simulink model "Michaels_CVModel_fast8"  (R2020a)
settings: Solver=ode23  StartTime=0.0  StopTime=30  RelTol=1e-2  EnableMultiTasking=on
model workspace (MAT data in the model file):
  Eao = 1.88
  Eesla = 0.58
  Eeslvf = 5.2
  Eesra = 0.63
  Eesrvf = 1.75
  Emaxspt = 48.75
  Epa = 0.15
  Epu = 0.04
  Esa = 0.37
  Esv = 0.013
  Evc = 0.03
  GpLV = 0
  GpRR = 11
  GpRV = 0
  GpRsa = 0
  GpV0 = 0
  GsLV = 0.007
  GsRR = 11
  GsRV = 0.022
  GsRsa = -0.05
  GsV0 = 31
  Ka = 4.4
  Lao = 0.0022
  Lav = 0.000354
  Lmt = 7.697e-05
  Lpa = 7.697e-05
  Lpv = 0.0001043
  Ltc = 8.009e-05
  P0la = 0.5
  P0lvf = 0.98
  P0pcd = 0.5
  P0ra = 0.5
  P0rvf = 0.91
  P0spt = 0.46
  PV.AO.p = [0 20 40 60 80 100 120 140 160 180]
  PV.AO.v = [52.2 64.3 81.3 102.1 130 150.7 163.1 173.9 179 183.6]
  PVao = [327.9; 100.9]
  Rao = 0.28
  Rav = 0.02
  Rla2pu = 0.5
  Rmt = 0.01
  Rpa = 0.12
  Rpa_Vals = 0.12
  Rpu = 0.006
  Rpv = 0.02
  Rra = 0.012
  Rsa = 0.74
  Rsv = 0.12
  Rtc = 0.01
  Tc = 1
  Tsys0 = 0.6
  V0la = 30
  V0lvf = 45
  V0pcd = 200
  V0ra = 25
  V0rvf = 50
  V0spt = 10
  Vdla = 15
  Vdlvf = 16
  Vdra = 15
  Vdrvf = 40
  Vdspt = 10
  Vlv0 = 100
  Vperi = 51
  Vrv0 = 105
  Vuao = 260.8
  Vupa = 91
  Vupu = 132
  Vusa = 287.4
  Vusv = 1976.1
  Vuvc = 136.17
  amin = -2
  artBrLVcontConti = []
  artBrLVcontDigi = [0 0 0 0 0 0 0 0 0 0 0 0 ... (240 elements, 1x240)]
  artBrRRConti = []
  artBrRRDigi = [0 0 0 0 0 0 0 0 0 0 1.57142857143 3.14285714286 ... (240 elements, 1x240)]
  artBrRVcontConti = []
  artBrRVcontDigi = [0 0 0 0 0 0 0 0 0 0 0 0 ... (240 elements, 1x240)]
  artBrRsaConti = []
  artBrRsaDigi = [0 0 0 0 0 0 0 0 0 0 0 0 ... (480 elements, 1x480)]
  artBrV0Conti = []
  artBrV0Digi = [0 0 0 0 0 0 0 0 0 0 0 0 ... (640 elements, 1x640)]
  atriumA = 1
  baroSampFreq = 16
  cP0la = 0.5
  cP0lvf = 0.98
  cP0ra = 0.5
  cP0rvf = 0.91
  cT = 1
  cVtotal = 5400
  clambdala = 0.13
  clambdalvf = 0.028
  clambdara = 0.13
  clambdarvf = 0.028
  deac = 0.0004
  ksys = 0.075
  lambdala = 0.065
  lambdalvf = 0.042
  lambdapcd = 0.005
  lambdara = 0.065
  lambdarvf = 0.028
  lambdaspt = 0.4
  pThor = 0
  params.lvf.lambda = 0.028
  params.lvf.P0 = 0.98
  params.lvf.V0 = 40
  params.lvf.Ees = 3.54
  params.lvf.Vd = 16.77
  params.rvf.lambda = 0.028
  params.rvf.P0 = 0.91
  params.rvf.V0 = 50
  params.rvf.Ees = 1.75
  params.rvf.Vd = 40.8
  params.la.lambda = 0.025
  params.la.P0 = 0.5
  params.la.V0 = 20
  params.la.Ees = 0.2
  params.la.Vd = 10
  params.ra.lambda = 0.025
  params.ra.P0 = 0.5
  params.ra.V0 = 20
  params.ra.Ees = 0.2
  params.ra.Vd = 10
  params.ventricle.Tsys0 = 0.6
  params.ventricle.ksys = 0.075
  params.ventricle.k1 = 0.5
  params.ventricle.k2 = 0.5
  params.atrium.A = 1
  params.Lao = 0.0001043
  params.Lpa = 7.697e-05
  params.Rtc = 0.01
  params.Rpv = 0.02
  params.Rmt = 0.01
  params.Rav = 0.02
  params.Rao = 0.2
  params.Rsa = 0.74
  params.Rsv = 0.12
  params.Rra = 0.012
  params.Rpa = 0.12
  params.Rpu = 0.006
  params.ao.E = 1.04
  params.ao.V0 = 230.880769231
  params.sa.E = 0.37
  params.sa.V0 = 231.04
  params.sv.E = 0.013
  params.sv.V0 = 1976.1
  params.vc.E = 0.03
  params.vc.V0 = 136.17
  params.pa.E = 0.15
  params.pa.V0 = 91.67
  params.pu.E = 0.04
  params.pu.V0 = 132.39
  params.cVtotal = 5300
  sampleTime = 0.005
  svcPressureChange_MCS = 0
  svrMult = 1
  tStepOn = 1000000000
  t_baroOn = 1000000
  t_testBed_start = 1000000
  venk1 = 0.5
  venk2 = 0.5
undefined symbols (not defined in the file): dfilt
libraries: simulink x85, fl_lib x39, nesl_utility x24, cstblocks x9, dspstat3 x9, dspobslib x5, SimscapeFluids_lib x5, sh_lib x1
(part 1 of 5)
settings Model: MinMaxOverflowLogging=ForceOff  SimulationMode=accelerator  Creator=Michael  LastModifiedBy=mangoez
settings DataIOCC: InitialState=xStart  MaxDataPoints=1  SaveFormat=Array  SaveOutput=off  SaveTime=off  ReturnWorkspaceOutputs=off  DatasetSignalFormat=timetable
settings OptimizationCC: DefaultParameterBehavior=Inlined  ExpressionDepthLimit=2147483647  LifeSpan=inf
settings DebuggingCC: SolverPrmCheckMsg=warning  FcnCallInpInsideContextMsg=warning  ModelReferenceExtraNoncontSigs=warning  StateNameClashWarn=warning  SFUnexpectedBacktrackingDiag=warning  SFNoUnconditionalDefaultTransitionDiag=warning  ArithmeticOperatorsInVariantConditions=warning
settings HardwareCC: ProdBitPerPointer=32  ProdBitPerSizeT=32  ProdBitPerPtrDiffT=32  ProdLargestAtomicFloat=None  ProdIntDivRoundTo=Undefined  ProdEndianess=Unspecified  ProdWordSize=32  ProdHWDeviceType=32-bit Generic
settings ModelReferenceCC: ModelReferenceNumInstancesAllowed=Single  ModelReferenceMinAlgLoopOccurrences=on  PropagateSignalLabelsOutOfModel=off
settings SFSimCC: SimUseLocalCustomCode=off  SimParseCustomCode=off  CustomCodeUndefinedFunction=UseInterfaceOnly
settings RTWCC: RTWUseLocalCustomCode=off
settings CodeAppCC: StateflowObjectComments=on
settings GRTTargetCC: TargetLangStandard=C89/C90 (ANSI)  CombineOutputUpdateFcns=off  GRTInterface=on
settings ConfigComp: CovMetricSettings=dw  CovHtmlReporting=on  CovSaveCumulativeToWorkspaceVar=on  CovSaveSingleToWorkspaceVar=on  CovExternalEMLEnable=off

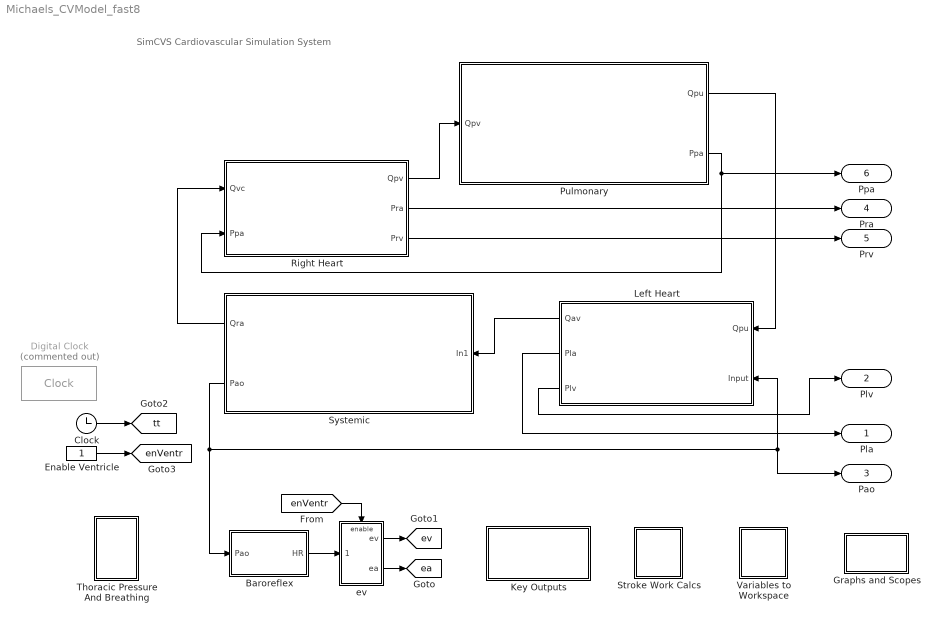
== system Michaels_CVModel_fast8 ==
  note: SimCVS
      | Cardiovascular Simulation System
  Baroreflex : Subsystem
  Clock : Clock
  Digital Clock : DigitalClock  Commented=on  SampleTime=0.001
  Enable Ventricle : Constant
  Graphs and Scopes : Subsystem
  Key Outputs : Subsystem
  Left Heart : Subsystem
      mask Display:
      | disp('LEFT HEART')
      | port_label('output',1,'Qav')
      | port_label('output',2,'Pla')
      | port_label('output',3,'Plv')
      | port_label('input',1,'Qpu')
      | port_label('input',2,'Pao')
  Pulmonary : Subsystem
      mask Display:
      | disp('PULMONARY CIRCULATORY SYSTEM')
      | port_label('output',1,'Qpu')
      | port_label('output',2,'Ppa')
      | port_label('input',1,'Qpv')
  Right Heart : Subsystem
      mask Display:
      | disp('RIGHT HEART')
      | port_label('output',1,'Qpv')
      | port_label('output',2,'Pra')
      | port_label('output',3,'Prv')
      | port_label('input',1,'Qvc')
      | port_label('input',2,'Ppa')
  Stroke Work Calcs : Subsystem
  Systemic : Subsystem
      mask Display:
      | disp('SYSTEMIC CIRULATORY SYSTEM')
      | port_label('output', 1, 'Qra')
      | port_label('output', 2, 'Pao')
      | port_label('input', 1, 'Qav')
  Thoracic Pressure And Breathing : Subsystem
  Variables to Workspace : Subsystem
  ev : Subsystem
  Pla : Outport
  Plv : Outport  Port=2
  Pao : Outport  Port=3
  Pra : Outport  Port=4
  Prv : Outport  Port=5
  Ppa : Outport  Port=6
  tag scope: ea=global, enVentr=global, ev=global, tt=global
  wires:
  Left Heart/1(Qav) -> Systemic/1(In1)
  Systemic/1(Qra) -> Right Heart/1(Qvc)
  Left Heart/2(Pla) -> Pla/1
  Pulmonary/2(Ppa) -> Right Heart/2(Ppa), Ppa/1
  Right Heart/2(Pra) -> Pra/1
  Right Heart/3(Prv) -> Prv/1
  [enVentr] -> ev/Enable
  ev/2(ea) -> [ea]
  Clock/1 -> [tt]
  ev/1(ev) -> [ev]
  Baroreflex/1(HR) -> ev/1(HR in)
  Enable Ventricle/1 -> [enVentr]
  Right Heart/1(Qpv) -> Pulmonary/1(Qpv)
  Pulmonary/1(Qpu) -> Left Heart/1(Qpu)
  Systemic/2(Pao) -> Left Heart/2(Input), Pao/1, Baroreflex/1(Pao)
  Left Heart/3(Plv) -> Plv/1

== system Michaels_CVModel_fast8/Baroreflex ==
  Pao : Inport
  Baroreflex Heldt : Subsystem  Commented=on  TreatAsAtomicUnit=on
  Baroreflex Heldt cont : Subsystem  Commented=on  TreatAsAtomicUnit=on
  Baroreflex Lu : Subsystem  Commented=on  TreatAsAtomicUnit=on
  Baroreflex Off On : Constant  SampleTime=0.001
  Compare To Constant : simulink/Logic and Bit Operations/Compare To Constant  relop===  const=1  OutDataTypeStr=uint8
  Compare To Constant1 : simulink/Logic and Bit Operations/Compare To Constant  Commented=on  relop===  const=2  OutDataTypeStr=uint8
  Compare To Constant2 : simulink/Logic and Bit Operations/Compare To Constant  Commented=on  relop===  const=3  OutDataTypeStr=uint8
  Compare To Constant3 : simulink/Logic and Bit Operations/Compare To Constant  Commented=on  relop===  const=4  OutDataTypeStr=uint8
  Constant : Constant  Value=0
  Demux : Demux  Description=0  Outputs=5
  From44 : From  Commented=on  GotoTag=Vsa  TagVisibility=global
  Multiport Switch : MultiPortSwitch  Inputs=4
  Multiport Switch1 : MultiPortSwitch  Inputs=4
  Multiport Switch2 : MultiPortSwitch  Inputs=4
  No Baroreflex : Subsystem  TreatAsAtomicUnit=on
  To Workspace1 : ToWorkspace  Commented=on  VariableName=aFcon  SampleTime=0.005
  To Workspace2 : ToWorkspace  Commented=on  VariableName=HeartRate  SampleTime=0.005
  To Workspace3 : ToWorkspace  Commented=on  VariableName=aFconRV  SampleTime=0.005
  To Workspace4 : ToWorkspace  Commented=on  VariableName=Vusv  SampleTime=0.005
  HR : Outport
  tag scope: HeartRate=global, Rsa=global, Vusv=global, aFconLV=global, aFconRV=global
  wires:
  Multiport Switch/1 -> Compare To Constant1/1, Compare To Constant/1, Compare To Constant2/1, Compare To Constant3/1
  Compare To Constant/1 -> No Baroreflex/Enable
  Compare To Constant1/1 -> Baroreflex Lu/Enable
  Compare To Constant2/1 -> Baroreflex Heldt/Enable
  Multiport Switch1/1 -> Baroreflex Heldt/1(Pao), Baroreflex Lu/1(Pao), Baroreflex Heldt cont/1(Pao)
  No Baroreflex/1(out) -> Multiport Switch2/2
  Baroreflex Lu/1(out) -> Multiport Switch2/3
  Baroreflex Heldt/1(out) -> Multiport Switch2/4
  From44/1 -> Baroreflex Lu/2(Vsa)
  Multiport Switch2/1 -> Demux/1
  Demux/1 -> [HeartRate], HR/1, To Workspace2/1  "HR"
  Demux/2 -> [aFconLV], To Workspace1/1
  Demux/3 -> [aFconRV], To Workspace3/1
  Baroreflex Heldt cont/1(out) -> Multiport Switch2/5
  Compare To Constant3/1 -> Baroreflex Heldt cont/Enable
  Demux/5 -> [Vusv], To Workspace4/1
  Baroreflex Off On/1 -> Multiport Switch2/1, Multiport Switch1/1, Multiport Switch/5, Multiport Switch/4, Multiport Switch/3, Multiport Switch/2, Multiport Switch/1
  Pao/1 -> Multiport Switch1/5, Multiport Switch1/4, Multiport Switch1/3
  Constant/1 -> Multiport Switch1/2
  Demux/4 -> [Rsa]  "Rsa"

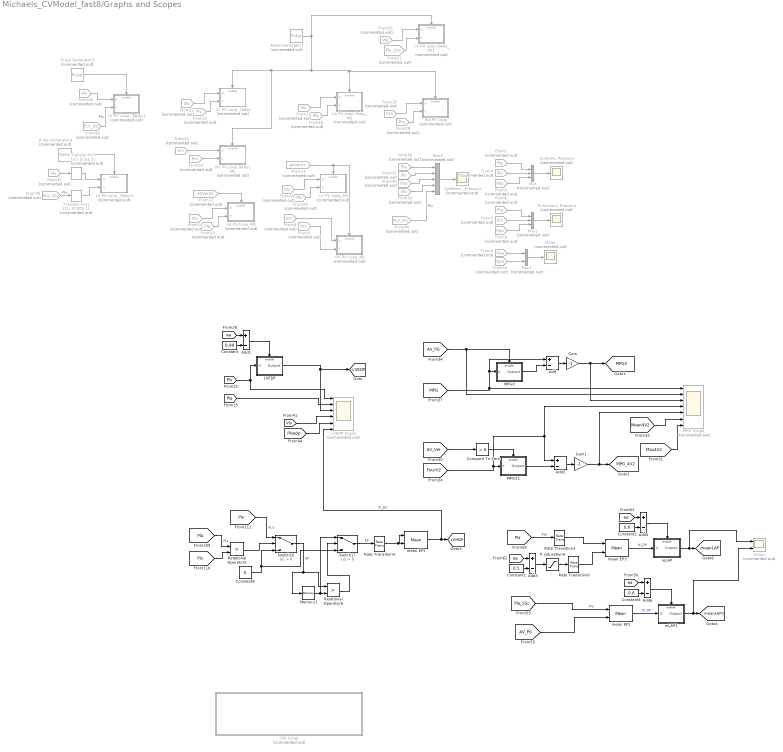
== system Michaels_CVModel_fast8/Graphs and Scopes ==
  Add{,1..4,6} (6 alike) : Sum  Inputs=+-
  Compare To Zero : simulink/Logic and Bit Operations/Compare To Zero  relop=>  OutDataTypeStr=boolean
  Constant : Constant  Value=0.99
  Constant1 : Constant  Value=0.5
  Constant2 : Constant  Value=0.6
  Constant4 : Constant  Value=0.6
  Constant8 : Constant  Value=0
  Flows : Scope  Commented=on
  From{1,13,16,36} (4 alike) : From  Commented=on  GotoTag=Pla  TagVisibility=global
      settings: CloseFcn=tagdialog Close
  From10 : From  Commented=on  GotoTag=Qpa  TagVisibility=global
      settings: CloseFcn=tagdialog Close
  From11 : From  Commented=on  GotoTag=enVentr  TagVisibility=global
  From12 : From  Commented=on  GotoTag=enVentr  TagVisibility=global
  From14 : From  Commented=on  GotoTag=Vla  TagVisibility=global
      settings: CloseFcn=tagdialog Close
  From17 : From  Commented=on  GotoTag=Vla  TagVisibility=global
      settings: CloseFcn=tagdialog Close
  From18 : From  Commented=on  GotoTag=Pra  TagVisibility=global
      settings: CloseFcn=tagdialog Close
  From19 : From  Commented=on  GotoTag=Vra  TagVisibility=global
      settings: CloseFcn=tagdialog Close
  From2 : From  Commented=on  GotoTag=Prv  TagVisibility=global
      settings: CloseFcn=tagdialog Close
  From20 : From  Commented=on  GotoTag=Prv  TagVisibility=global
      settings: CloseFcn=tagdialog Close
  From{4,21,37,43} (4 alike) : From  Commented=on  GotoTag=Plv  TagVisibility=global
      settings: CloseFcn=tagdialog Close
  From{22,28,33,39,54} (5 alike) : From  Commented=on  GotoTag=Vlv  TagVisibility=global
      settings: CloseFcn=tagdialog Close
  From23 : From  Commented=on  GotoTag=Vrv  TagVisibility=global
      settings: CloseFcn=tagdialog Close
  From29 : From  Commented=on  GotoTag=PLV_SSc  TagVisibility=global
      settings: CloseFcn=tagdialog Close
  From3 : From  Commented=on  GotoTag=Vrv  TagVisibility=global
      settings: CloseFcn=tagdialog Close
  From35 : From  Commented=on  GotoTag=PLV_SSc  TagVisibility=global
      settings: CloseFcn=tagdialog Close
  From38 : From  Commented=on  GotoTag=Pao  TagVisibility=global
      settings: CloseFcn=tagdialog Close
  From40 : From  Commented=on  GotoTag=PLV_SSc  TagVisibility=global
      settings: CloseFcn=tagdialog Close
  From5 : From  Commented=on  GotoTag=Pao  TagVisibility=global
      settings: CloseFcn=tagdialog Close
  From51 : From  Commented=on  GotoTag=Pla_SSc  TagVisibility=global
      settings: CloseFcn=tagdialog Close
  From52 : From  Commented=on  GotoTag=Vla  TagVisibility=global
      settings: CloseFcn=tagdialog Close
  From6 : From  Commented=on  GotoTag=Pra  TagVisibility=global
      settings: CloseFcn=tagdialog Close
  From7 : From  Commented=on  GotoTag=Prv  TagVisibility=global
      settings: CloseFcn=tagdialog Close
  From8 : From  Commented=on  GotoTag=Ppa  TagVisibility=global
      settings: CloseFcn=tagdialog Close
  From9 : From  Commented=on  GotoTag=Qsa  TagVisibility=global
      settings: CloseFcn=tagdialog Close
  Gain : Gain  Gain=-1
  Gain1 : Gain  Gain=-1
  LA PV Loop Delay_MS : Subsystem  Commented=on  TreatAsAtomicUnit=on
  LA PV Loop Delay_MS1 : Subsystem  Commented=on  TreatAsAtomicUnit=on
  LA PV Loop_MS : Subsystem  Commented=on  TreatAsAtomicUnit=on
  LV PV Loop _Delay : Subsystem  Commented=on  TreatAsAtomicUnit=on
  LV PV Loop _Delay1 : Subsystem  Commented=on  TreatAsAtomicUnit=on
  LV PV Loop _Delay2 : Subsystem  Commented=on  TreatAsAtomicUnit=on
  LV PV Loop_MS : Subsystem  Commented=on  TreatAsAtomicUnit=on
  LVEDP : Subsystem  TreatAsAtomicUnit=on
  LVEDP Scope : Scope  Commented=on  NumInputPorts=6
  MPG Scope : Scope  Commented=on  NumInputPorts=7
  MPGX : Subsystem  TreatAsAtomicUnit=on
  MPGX1 : Subsystem  TreatAsAtomicUnit=on
  Memory1 : Memory
  Mux : Mux  Commented=on  Inputs=3
  Mux1 : Mux  Commented=on  Inputs=3
  Mux2 : Mux  Commented=on  Inputs=2
  Mux3 : Mux  Commented=on  Inputs=5
  P saturation4 : Saturate  UpperLimit=inf  LowerLimit=0
  Pulmonary Pressure : Scope  Commented=on
  Pulse Generator2 : DiscretePulseGenerator  Commented=on  PulseType=Time based  Period=20  PulseWidth=99  PhaseDelay=27.7
  Pulse Generator3 : DiscretePulseGenerator  Commented=on  PulseType=Time based  Period=20  PulseWidth=99  PhaseDelay=27.7
  Pulse Generator4 : DiscretePulseGenerator  Commented=on  PulseType=Time based  Period=20  PulseWidth=99  PhaseDelay=39.7
  RA PV Loop : Subsystem  Commented=on  TreatAsAtomicUnit=on
  RV PV Loop Delay_MS : Subsystem  Commented=on  TreatAsAtomicUnit=on
  RV PV Loop_MS : Subsystem  Commented=on  TreatAsAtomicUnit=on
  Rate Transition3 : RateTransition  OutPortSampleTime=0.001
  Rate Transition4 : RateTransition  OutPortSampleTime=0.001
  Rate Transition6 : RateTransition  OutPortSampleTime=0.001
  Relational Operator5 : RelationalOperator  Operator=>  OutDataTypeStr=boolean  ZeroCross=off  RndMeth=Simplest
  Relational Operator6 : RelationalOperator  Operator=>  OutDataTypeStr=boolean  ZeroCross=off  RndMeth=Simplest
  SW Scrap : Subsystem  Commented=on
  Scope : Scope  Commented=on  NumInputPorts=2
  Switch16 : Switch  Criteria=u2 > Threshold
  Switch17 : Switch  Criteria=u2 > Threshold
  Systemic Pressure : Scope  Commented=on
  Systemic _Pressure : Scope  Commented=on
  Transfer Fcn : TransferFcn  Commented=on  Denominator=[0.01 1]
  Transfer Fcn1 : TransferFcn  Commented=on  Denominator=[0.005 1]
  mLAP : Subsystem  TreatAsAtomicUnit=on
  mLAP1 : Subsystem  TreatAsAtomicUnit=on
  mean EP1 : dspstat3/Mean  run=on  reset_popup=Rising edge  directionMode=Each column  dimension=1  roiEnable=off  roiType=Rectangles  roiPortion=Entire ROI  roiOutput=Individual statistics for each ROI  roiFlag=off  roundingMode=Floor  overflowMode=off  outputDataTypeStr=Inherit: Same as accumulator  outputMin=[]  outputMax=[]  outputLastDataTypeStr=Inherit: Same as accumulator
  mean EP2 : dspstat3/Mean  run=on  reset_popup=Either edge  directionMode=Each column  dimension=1  roiEnable=off  roiType=Rectangles  roiPortion=Entire ROI  roiOutput=Individual statistics for each ROI  roiFlag=off  roundingMode=Floor  overflowMode=off  outputDataTypeStr=Inherit: Same as accumulator  outputMin=[]  outputMax=[]  outputLastDataTypeStr=Inherit: Same as accumulator
  mean EP3 : dspstat3/Mean  run=on  reset_popup=Falling edge  directionMode=Each column  dimension=1  roiEnable=off  roiType=Rectangles  roiPortion=Entire ROI  roiOutput=Individual statistics for each ROI  roiFlag=off  roundingMode=Floor  overflowMode=off  outputDataTypeStr=Inherit: Same as accumulator  outputMin=[]  outputMax=[]  outputLastDataTypeStr=Inherit: Same as accumulator
  tag scope: LVEDP=global, LVMDP=global, MPGX=global, MPG_4V2=global, meanLAP2=global, meanLAP=global
  wires:
  From1/1 -> Mux/1
  From4/1 -> Mux/2
  From5/1 -> Mux/3
  Mux/1 -> Systemic Pressure/1
  From6/1 -> Mux1/1
  From7/1 -> Mux1/2
  From8/1 -> Mux1/3
  Mux1/1 -> Pulmonary Pressure/1
  From9/1 -> Mux2/1
  From10/1 -> Mux2/2
  Mux2/1 -> Flows/1
  From3/1 -> RV PV Loop_MS/1(X)
  From2/1 -> RV PV Loop_MS/2(Y)
  From54/1 -> LV PV Loop_MS/1(X)
  From43/1 -> LV PV Loop_MS/2(Y)
  From11/1 -> LV PV Loop_MS/Enable, RV PV Loop_MS/Enable
  From14/1 -> LA PV Loop_MS/1(X)
  From12/1 -> LA PV Loop_MS/Enable
  From13/1 -> LA PV Loop_MS/2(Y)
  From16/1 -> LA PV Loop Delay_MS/2(Y)
  From17/1 -> LA PV Loop Delay_MS/1(X)
  From19/1 -> RA PV Loop/1(X)
  From18/1 -> RA PV Loop/2(Y)
  From22/1 -> LV PV Loop _Delay/1(X)
  From21/1 -> LV PV Loop _Delay/2(Y)
  From20/1 -> RV PV Loop Delay_MS/2(Y)
  From23/1 -> RV PV Loop Delay_MS/1(X)
  [AV_PG] -> MPG Scope/2, MPGX/Enable
  MPGX/1(Outport) -> Add/2
  LVEDP/1(Outport) -> [LVEDP], LVEDP Scope/3
  Gain/1 -> MPG Scope/3, [MPGX]
  Add/1 -> Gain/1
  [Plv] -> LVEDP/1(X), LVEDP Scope/1
  [MPG] -> MPG Scope/1, Add/1, MPGX/1(X)
  [Pla] -> LVEDP Scope/2
  Constant/1 -> Add1/2
  [ea] -> Add1/1
  Add1/1 -> LVEDP/Enable
  Pulse Generator3/1 -> LV PV Loop _Delay1/Enable
  From28/1 -> LV PV Loop _Delay1/1(X)
  From29/1 -> LV PV Loop _Delay1/2(Y)  "Plv"
  [Vlv] -> LVEDP Scope/4
  [Plvedp] -> LVEDP Scope/5
  [FourV2] -> MPGX1/1(X), MPG Scope/4, Add2/1
  Add2/1 -> Gain1/1
  Gain1/1 -> [MPG_4V2], MPG Scope/5
  MPGX1/1(Outport) -> Add2/2
  [AV_Vel] -> Compare To Zero/1
  [Max4V2] -> MPG Scope/7
  Mux3/1 -> Systemic _Pressure/1
  From38/1 -> Mux3/3
  From37/1 -> Mux3/2
  From36/1 -> Mux3/1
  From39/1 -> Mux3/4
  [Plv] -> Relational Operator5/2
  Relational Operator6/1 -> Switch17/2
  Rate Transition4/1 -> mean EP2/1, mean EP2/2
  Memory1/1 -> Switch17/1, Relational Operator6/2
  Switch16/1 -> Memory1/1, Relational Operator6/1  "EP"
  Switch17/1 -> Rate Transition4/1  "EP"
  [Pla] -> Relational Operator5/1  "Pla"
  [Plv] -> Switch16/1  "PLV"
  Constant8/1 -> Switch17/3, Switch16/3
  Relational Operator5/1 -> Switch16/2
  mean EP2/1 -> LVEDP Scope/6, [LVMDP]  "M_DP"
  Compare To Zero/1 -> MPGX1/Enable
  [Mean4V2] -> MPG Scope/6
  From35/1 -> Transfer Fcn1/1  "Plv"
  From33/1 -> Transfer Fcn/1
  Pulse Generator4/1 -> LV PV Loop _Delay2/Enable
  Transfer Fcn/1 -> LV PV Loop _Delay2/1(X)
  Transfer Fcn1/1 -> LV PV Loop _Delay2/2(Y)
  From40/1 -> Mux3/5  "Plv"
  [Pla] -> Rate Transition3/1  "Pla"
  mean EP3/1 -> mLAP/1(X)  "M_DP"
  Rate Transition3/1 -> mean EP3/1
  Constant1/1 -> Add3/2
  [ea] -> Add3/1
  Add3/1 -> P saturation4/1
  P saturation4/1 -> Rate Transition6/1
  Rate Transition6/1 -> mean EP3/2
  Add4/1 -> mLAP/Enable
  [ea] -> Add4/1
  mLAP/1(Outport) -> Scope/1, [meanLAP]
  Constant2/1 -> Add4/2
  Pulse Generator2/1 -> RV PV Loop Delay_MS/Enable, LV PV Loop _Delay/Enable, LA PV Loop Delay_MS/Enable, RA PV Loop/Enable, LA PV Loop Delay_MS1/Enable
  From52/1 -> LA PV Loop Delay_MS1/1(X)
  From51/1 -> LA PV Loop Delay_MS1/2(Y)
  Constant4/1 -> Add6/2
  mLAP1/1(Outport) -> Scope/2, [meanLAP2]
  [ea] -> Add6/1
  Add6/1 -> mLAP1/Enable
  mean EP1/1 -> mLAP1/1(X)  "M_DP"
  [Pla_SSc] -> mean EP1/1  "Pla"
  [AV_PG] -> mean EP1/2
